simulink model "simulacion2025"  (R2025a)
settings: Solver=VariableStepAuto  StartTime=0.0  StopTime=30  MaxStep=1e-3  RelTol=1e-4
values from neighbouring files (symbols this model uses):
  B = 0.3441    [datos_planta.m]
  Fg = 0.6263    [datos_planta.m]
  J = 0.0112    [datos_planta.m]
  Jb = (305490.04e-12)*0.1    (= 3.0549004e-08)    [datos_planta.m]
  Jv = 13576.379e-12    (= 1.3576379e-08)    [datos_planta.m]
  Ka = 0.2335    [datos_planta.m]
  Km = 0.147    [datos_planta.m]
  L = 0.52    [datos_planta.m]
  m = 0.06385    [datos_planta.m]
  R = 1.6    [datos_planta.m]
  Rr = 21    [datos_planta.m]
  Tm = 0.41    [datos_planta.m]
undefined symbols (not defined in the file or in its folder): x
libraries: slpidlib x31
(part 2 of 2)

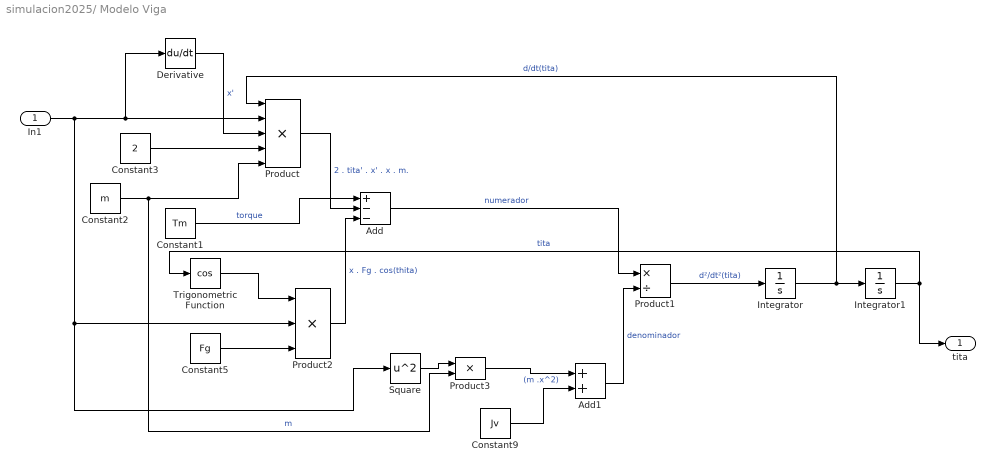
== system simulacion2025/ Modelo Viga ==
  In1 : Inport
  Add : Sum  Inputs=+--
  Add1 : Sum
  Constant1 : Constant  Value=Tm
  Constant2 : Constant  Value=m
  Constant3 : Constant  Value=2
  Constant5 : Constant  Value=Fg
  Constant9 : Constant  Value=Jv
  Derivative : Derivative
  Integrator : Integrator
  Integrator1 : Integrator
  Product : Product  Inputs=5
  Product1 : Product  Inputs=*/
  Product2 : Product  Inputs=3
  Product3 : Product
  Square : Math  Operator=square
  Trigonometric Function : Trigonometry  Operator=cos
  tita : Outport
  wires:
  Product1/1 -> Integrator/1  "d²/dt²(tita)"
  Integrator1/1 -> tita/1, Trigonometric Function/1  "tita"
  Integrator/1 -> Product/1, Integrator1/1  "d/dt(tita)"
  Product/1 -> Add/2  "2 . tita' . x' . x . m."
  Constant2/1 -> Product3/2, Product/5  "m"
  Constant3/1 -> Product/4
  Derivative/1 -> Product/3  "x'"
  Trigonometric Function/1 -> Product2/1
  In1/1 -> Product2/2, Square/1, Derivative/1, Product/2
  Constant5/1 -> Product2/3
  Product2/1 -> Add/3  "x . Fg . cos(thita)"
  Add/1 -> Product1/1  "numerador"
  Constant1/1 -> Add/1  "torque"
  Square/1 -> Product3/1
  Product3/1 -> Add1/1  "(m .x^2)"
  Add1/1 -> Product1/2  "denominador"
  Constant9/1 -> Add1/2

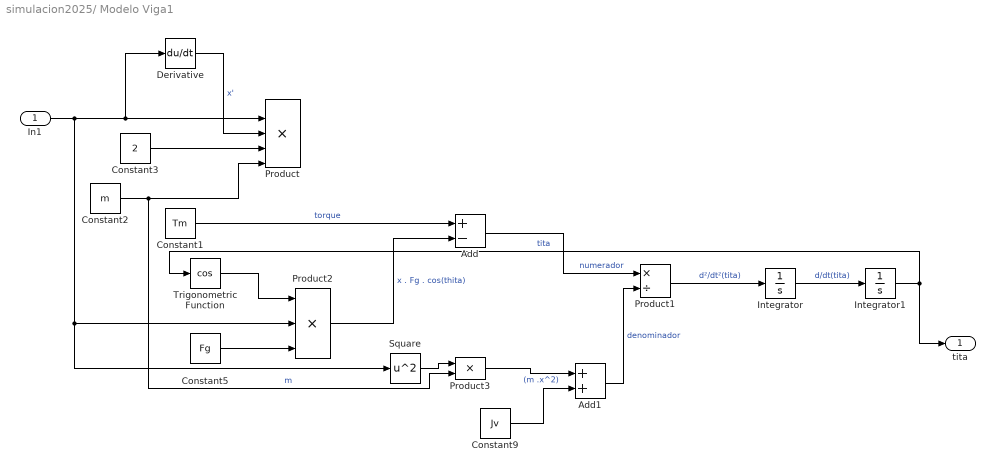
== system simulacion2025/ Modelo Viga1 ==
  In1 : Inport
  Add : Sum  Inputs=+-
  Add1 : Sum
  Constant1 : Constant  Value=Tm
  Constant2 : Constant  Value=m
  Constant3 : Constant  Value=2
  Constant5 : Constant  Value=Fg
  Constant9 : Constant  Value=Jv
  Derivative : Derivative
  Integrator : Integrator
  Integrator1 : Integrator
  Product : Product  Inputs=5
  Product1 : Product  Inputs=*/
  Product2 : Product  Inputs=3
  Product3 : Product
  Square : Math  Operator=square
  Trigonometric Function : Trigonometry  Operator=cos
  tita : Outport
  wires:
  Product1/1 -> Integrator/1  "d²/dt²(tita)"
  Integrator1/1 -> tita/1, Trigonometric Function/1  "tita"
  Integrator/1 -> Integrator1/1  "d/dt(tita)"
  Constant2/1 -> Product3/2, Product/5  "m"
  Constant3/1 -> Product/4
  Derivative/1 -> Product/3  "x'"
  Trigonometric Function/1 -> Product2/1
  In1/1 -> Product2/2, Square/1, Derivative/1, Product/2
  Constant5/1 -> Product2/3
  Constant1/1 -> Add/1  "torque"
  Square/1 -> Product3/1
  Product3/1 -> Add1/1  "(m .x^2)"
  Add1/1 -> Product1/2  "denominador"
  Constant9/1 -> Add1/2
  Product2/1 -> Add/2  "x . Fg . cos(thita)"
  Add/1 -> Product1/1  "numerador"

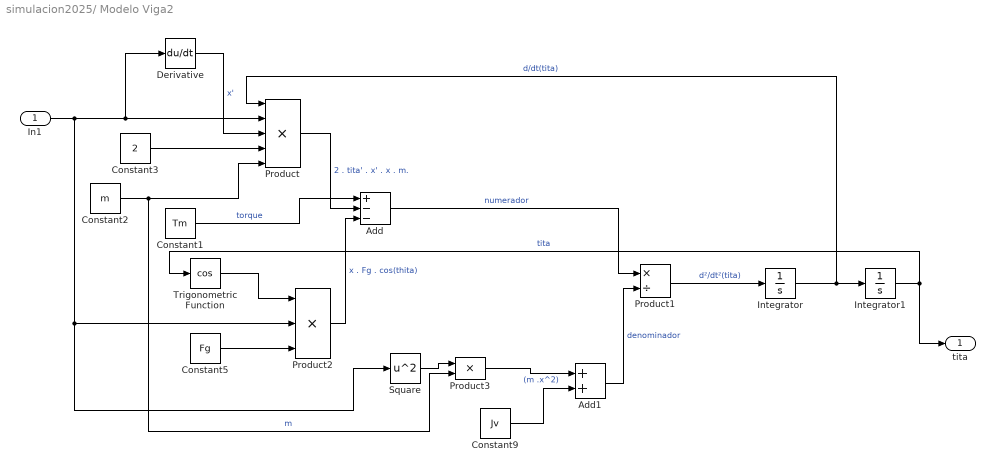
== system simulacion2025/ Modelo Viga2 ==
  In1 : Inport
  Add : Sum  Inputs=+--
  Add1 : Sum
  Constant1 : Constant  Value=Tm
  Constant2 : Constant  Value=m
  Constant3 : Constant  Value=2
  Constant5 : Constant  Value=Fg
  Constant9 : Constant  Value=Jv
  Derivative : Derivative
  Integrator : Integrator
  Integrator1 : Integrator
  Product : Product  Inputs=5
  Product1 : Product  Inputs=*/
  Product2 : Product  Inputs=3
  Product3 : Product
  Square : Math  Operator=square
  Trigonometric Function : Trigonometry  Operator=cos
  tita : Outport
  wires:
  Product1/1 -> Integrator/1  "d²/dt²(tita)"
  Integrator1/1 -> tita/1, Trigonometric Function/1  "tita"
  Integrator/1 -> Product/1, Integrator1/1  "d/dt(tita)"
  Product/1 -> Add/2  "2 . tita' . x' . x . m."
  Constant2/1 -> Product3/2, Product/5  "m"
  Constant3/1 -> Product/4
  Derivative/1 -> Product/3  "x'"
  Trigonometric Function/1 -> Product2/1
  In1/1 -> Product2/2, Square/1, Derivative/1, Product/2
  Constant5/1 -> Product2/3
  Product2/1 -> Add/3  "x . Fg . cos(thita)"
  Add/1 -> Product1/1  "numerador"
  Constant1/1 -> Add/1  "torque"
  Square/1 -> Product3/1
  Product3/1 -> Add1/1  "(m .x^2)"
  Add1/1 -> Product1/2  "denominador"
  Constant9/1 -> Add1/2

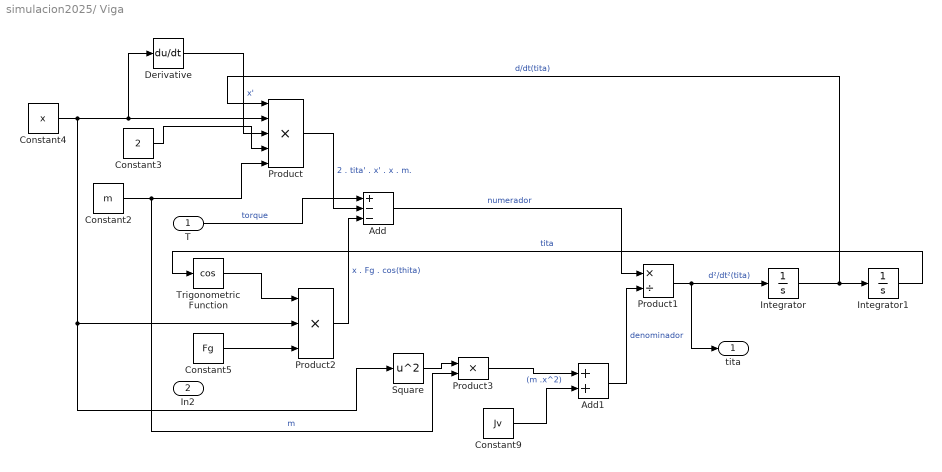
== system simulacion2025/ Viga ==
  T : Inport
  In2 : Inport  Port=2
  Add : Sum  Inputs=+--
  Add1 : Sum
  Constant2 : Constant  Value=m
  Constant3 : Constant  Value=2
  Constant4 : Constant  Value=x
  Constant5 : Constant  Value=Fg
  Constant9 : Constant  Value=Jv
  Derivative : Derivative
  Integrator : Integrator
  Integrator1 : Integrator
  Product : Product  Inputs=5
  Product1 : Product  Inputs=*/
  Product2 : Product  Inputs=3
  Product3 : Product
  Square : Math  Operator=square
  Trigonometric Function : Trigonometry  Operator=cos
  tita : Outport
  wires:
  Product1/1 -> tita/1, Integrator/1  "d²/dt²(tita)"
  Integrator1/1 -> Trigonometric Function/1  "tita"
  Integrator/1 -> Product/1, Integrator1/1  "d/dt(tita)"
  Product/1 -> Add/2  "2 . tita' . x' . x . m."
  Constant2/1 -> Product3/2, Product/5  "m"
  Constant3/1 -> Product/4
  Derivative/1 -> Product/3  "x'"
  Trigonometric Function/1 -> Product2/1
  Constant4/1 -> Product2/2, Square/1, Derivative/1, Product/2
  Constant5/1 -> Product2/3
  Product2/1 -> Add/3  "x . Fg . cos(thita)"
  Add/1 -> Product1/1  "numerador"
  T/1 -> Add/1  "torque"
  Square/1 -> Product3/1
  Product3/1 -> Add1/1  "(m .x^2)"
  Add1/1 -> Product1/2  "denominador"
  Constant9/1 -> Add1/2

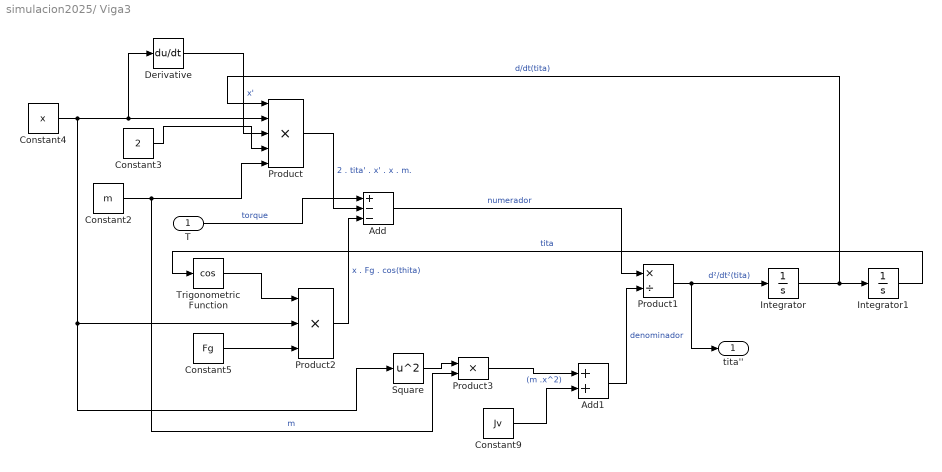
== system simulacion2025/ Viga3 ==
  T : Inport
  Add : Sum  Inputs=+--
  Add1 : Sum
  Constant2 : Constant  Value=m
  Constant3 : Constant  Value=2
  Constant4 : Constant  Value=x
  Constant5 : Constant  Value=Fg
  Constant9 : Constant  Value=Jv
  Derivative : Derivative
  Integrator : Integrator
  Integrator1 : Integrator
  Product : Product  Inputs=5
  Product1 : Product  Inputs=*/
  Product2 : Product  Inputs=3
  Product3 : Product
  Square : Math  Operator=square
  Trigonometric Function : Trigonometry  Operator=cos
  tita'' : Outport
  wires:
  Product1/1 -> tita''/1, Integrator/1  "d²/dt²(tita)"
  Integrator1/1 -> Trigonometric Function/1  "tita"
  Integrator/1 -> Product/1, Integrator1/1  "d/dt(tita)"
  Product/1 -> Add/2  "2 . tita' . x' . x . m."
  Constant2/1 -> Product3/2, Product/5  "m"
  Constant3/1 -> Product/4
  Derivative/1 -> Product/3  "x'"
  Trigonometric Function/1 -> Product2/1
  Constant4/1 -> Product2/2, Square/1, Derivative/1, Product/2
  Constant5/1 -> Product2/3
  Product2/1 -> Add/3  "x . Fg . cos(thita)"
  Add/1 -> Product1/1  "numerador"
  T/1 -> Add/1  "torque"
  Square/1 -> Product3/1
  Product3/1 -> Add1/1  "(m .x^2)"
  Add1/1 -> Product1/2  "denominador"
  Constant9/1 -> Add1/2

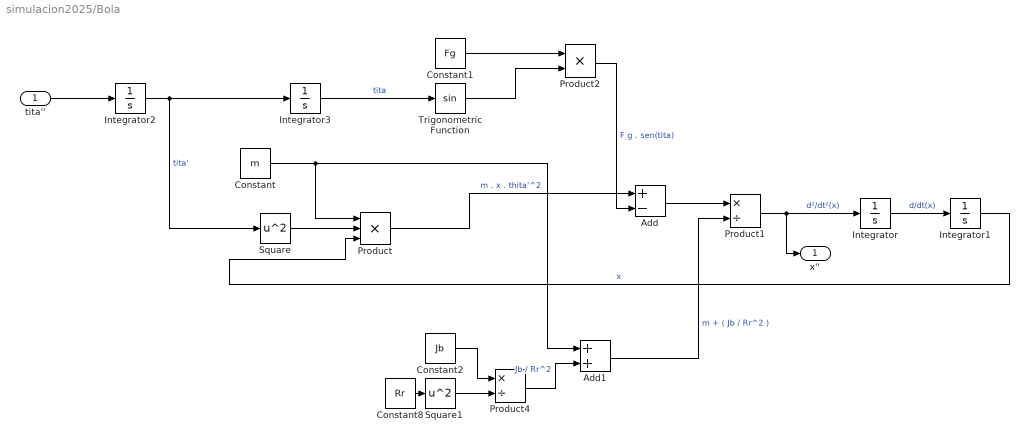
== system simulacion2025/Bola ==
  tita'' : Inport
  Add : Sum  Inputs=+-
  Add1 : Sum
  Constant : Constant  Value=m
  Constant1 : Constant  Value=Fg
  Constant2 : Constant  Value=Jb
  Constant8 : Constant  Value=Rr
  Integrator{,1..3} (4 alike) : Integrator
  Product : Product  Inputs=3
  Product1 : Product  Inputs=*/
  Product2 : Product
  Product4 : Product  Inputs=*/
  Square : Math  Operator=square
  Square1 : Math  Operator=square
  Trigonometric Function : Trigonometry
  x'' : Outport
  wires:
  Add/1 -> Product1/1
  Square/1 -> Product/2
  Integrator/1 -> Integrator1/1  "d/dt(x)"
  Integrator1/1 -> Product/3  "x"
  Integrator2/1 -> Square/1, Integrator3/1  "tita'"
  Product/1 -> Add/1  "m . x . thita'^2"
  Constant1/1 -> Product2/1
  Product2/1 -> Add/2  "F g . sen(tita)"
  tita''/1 -> Integrator2/1
  Product1/1 -> x''/1, Integrator/1  "d²/dt²(x)"
  Product4/1 -> Add1/2  "Jb / Rr^2"
  Constant2/1 -> Product4/1
  Constant/1 -> Add1/1, Product/1
  Square1/1 -> Product4/2
  Constant8/1 -> Square1/1
  Add1/1 -> Product1/2  "m + ( Jb / Rr^2 )"
  Integrator3/1 -> Trigonometric Function/1  "tita"
  Trigonometric Function/1 -> Product2/2

== system simulacion2025/Bola PosTaylor1 ==
  Constant2 : Constant  Value=Jb
  Constant6 : Constant  Value=-Fg
  Constant7 : Constant  Value=m
  Constant8 : Constant  Value=Rr
  Integrator1 : Integrator
  Integrator5 : Integrator
  Minus1 : Sum
  Product4 : Product  Inputs=*/
  Product7 : Product  Inputs=*/
  Square1 : Math  Operator=square
  Out1 : Outport
  wires:
  Constant6/1 -> Product7/1  "-Fg"
  Product7/1 -> Integrator5/1  "d²/dt²(x)"
  Integrator5/1 -> Integrator1/1  "delta.d(x)/dt"
  Integrator1/1 -> Out1/1  "d/dt(x)"
  Constant2/1 -> Product4/1
  Square1/1 -> Product4/2
  Constant8/1 -> Square1/1
  Product4/1 -> Minus1/2
  Constant7/1 -> Minus1/1
  Minus1/1 -> Product7/2

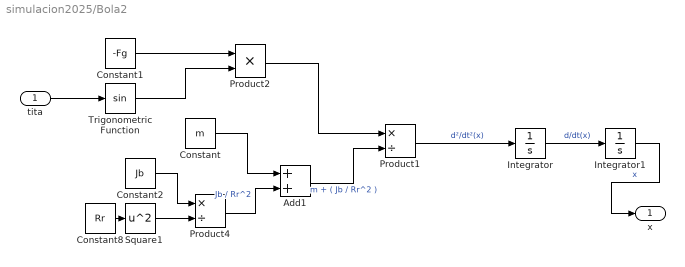
== system simulacion2025/Bola2 ==
  tita : Inport
  Add1 : Sum
  Constant : Constant  Value=m
  Constant1 : Constant  Value=-Fg
  Constant2 : Constant  Value=Jb
  Constant8 : Constant  Value=Rr
  Integrator : Integrator
  Integrator1 : Integrator
  Product1 : Product  Inputs=*/
  Product2 : Product
  Product4 : Product  Inputs=*/
  Square1 : Math  Operator=square
  Trigonometric Function : Trigonometry
  x : Outport
  wires:
  Product2/1 -> Product1/1
  Integrator/1 -> Integrator1/1  "d/dt(x)"
  Constant1/1 -> Product2/1
  Product1/1 -> Integrator/1  "d²/dt²(x)"
  Product4/1 -> Add1/2  "Jb / Rr^2"
  Constant2/1 -> Product4/1
  Constant/1 -> Add1/1
  Square1/1 -> Product4/2
  Constant8/1 -> Square1/1
  Add1/1 -> Product1/2  "m + ( Jb / Rr^2 )"
  tita/1 -> Trigonometric Function/1
  Trigonometric Function/1 -> Product2/2
  Integrator1/1 -> x/1  "x"

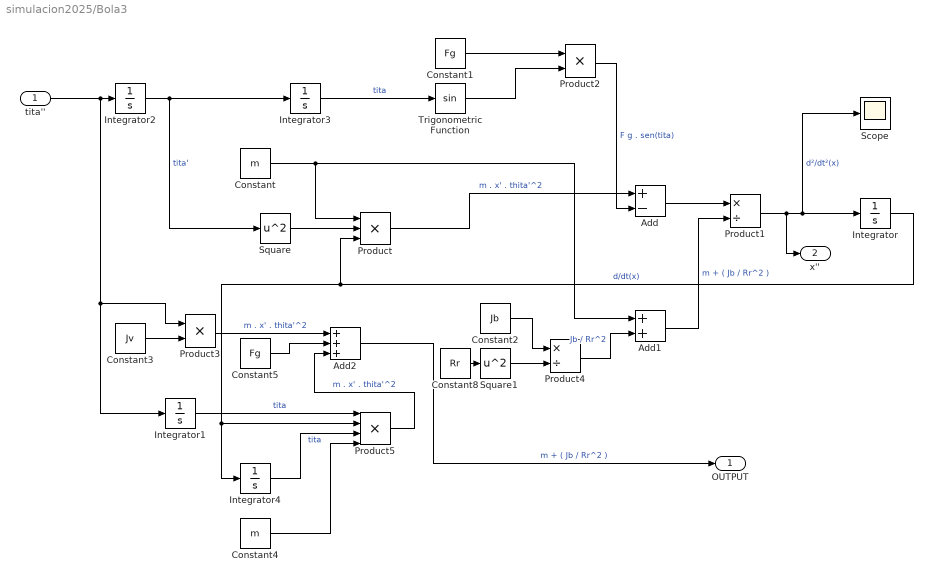
== system simulacion2025/Bola3 ==
  tita'' : Inport
  Add : Sum  Inputs=+-
  Add1 : Sum
  Add2 : Sum  Inputs=+++
  Constant : Constant  Value=m
  Constant1 : Constant  Value=Fg
  Constant2 : Constant  Value=Jb
  Constant3 : Constant  Value=Jv
  Constant4 : Constant  Value=m
  Constant5 : Constant  Value=Fg
  Constant8 : Constant  Value=Rr
  Integrator{,1..4} (5 alike) : Integrator
  Product : Product  Inputs=3
  Product1 : Product  Inputs=*/
  Product2 : Product
  Product3 : Product
  Product4 : Product  Inputs=*/
  Product5 : Product  Inputs=4
  Scope : Scope
      settings: ActiveDisplayYMinimum=-1.4787523574592083E+300  ActiveDisplayYMaximum=1.3308771217132878E+301  DataLoggingVariableName=ScopeData2
  Square : Math  Operator=square
  Square1 : Math  Operator=square
  Trigonometric Function : Trigonometry
  OUTPUT : Outport
  x'' : Outport  Port=2
  wires:
  Add/1 -> Product1/1
  Square/1 -> Product/2
  Integrator/1 -> Integrator4/1, Product5/2, Product/3  "d/dt(x)"
  Integrator2/1 -> Square/1, Integrator3/1  "tita'"
  Product/1 -> Add/1  "m . x' . thita'^2"
  Constant1/1 -> Product2/1
  Product2/1 -> Add/2  "F g . sen(tita)"
  Product1/1 -> x''/1, Scope/1, Integrator/1  "d²/dt²(x)"
  Product4/1 -> Add1/2  "Jb / Rr^2"
  Constant2/1 -> Product4/1
  Constant/1 -> Add1/1, Product/1
  Square1/1 -> Product4/2
  Constant8/1 -> Square1/1
  Add1/1 -> Product1/2  "m + ( Jb / Rr^2 )"
  Integrator3/1 -> Trigonometric Function/1  "tita"
  Trigonometric Function/1 -> Product2/2
  tita''/1 -> Integrator1/1, Product3/1, Integrator2/1
  Constant3/1 -> Product3/2
  Product3/1 -> Add2/1  "m . x' . thita'^2"
  Integrator1/1 -> Product5/1  "tita"
  Integrator4/1 -> Product5/3  "tita"
  Constant4/1 -> Product5/4
  Add2/1 -> OUTPUT/1  "m + ( Jb / Rr^2 )"
  Product5/1 -> Add2/3  "m . x' . thita'^2"
  Constant5/1 -> Add2/2

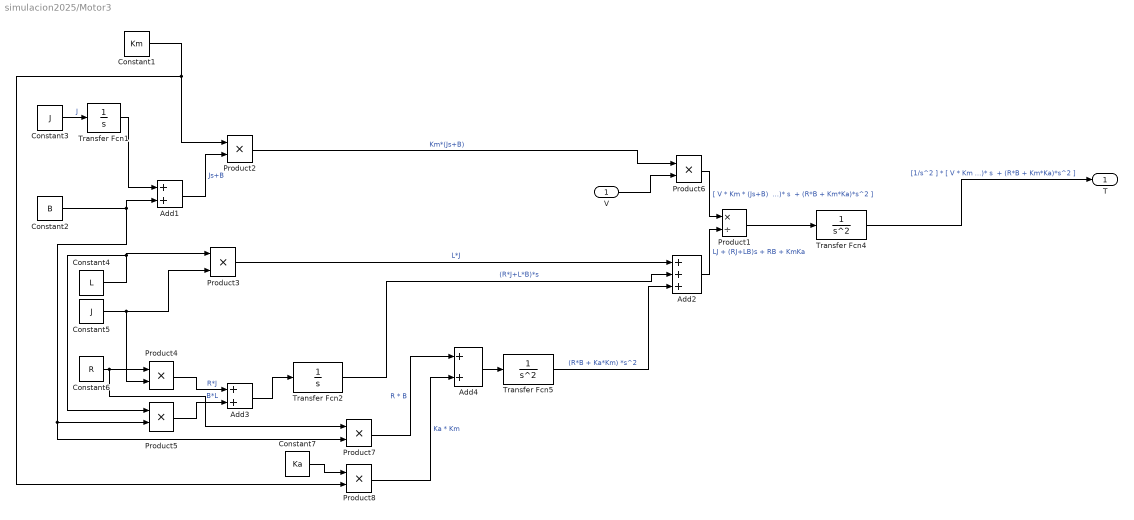
== system simulacion2025/Motor3 ==
  V : Inport
  Add1 : Sum
  Add2 : Sum  Inputs=+++
  Add3 : Sum
  Add4 : Sum
  Constant1 : Constant  Value=Km
  Constant2 : Constant  Value=B
  Constant3 : Constant  Value=J
  Constant4 : Constant  Value=L
  Constant5 : Constant  Value=J
  Constant6 : Constant  Value=R
  Constant7 : Constant  Value=Ka
  Product1 : Product  Inputs=*/
  Product{2..8} (7 alike) : Product
  Transfer Fcn1 : TransferFcn  Denominator=[0 1 0]
  Transfer Fcn2 : TransferFcn  Denominator=[0 1 0]
  Transfer Fcn4 : TransferFcn  Denominator=[1 0 0]
  Transfer Fcn5 : TransferFcn  Denominator=[1 0 0]
  T : Outport
  wires:
  Add1/1 -> Product2/2  "Js+B"
  Product2/1 -> Product6/1  "Km*(Js+B)"
  Constant5/1 -> Product3/2, Product4/2
  Constant4/1 -> Product5/1, Product3/1
  Product4/1 -> Add3/1  "R*J"
  Product5/1 -> Add3/2  "B*L"
  Add2/1 -> Product1/2  "LJ + (RJ+LB)s + RB + KmKa"
  Add3/1 -> Transfer Fcn2/1
  Transfer Fcn2/1 -> Add2/2  "(R*J+L*B)*s"
  Constant6/1 -> Product7/1, Product4/1
  Constant2/1 -> Add1/2, Product7/2, Product5/2
  Product7/1 -> Add4/1  "R * B"
  Constant7/1 -> Product8/1
  Constant1/1 -> Product2/1, Product8/2
  Product8/1 -> Add4/2  "Ka * Km"
  Constant3/1 -> Transfer Fcn1/1  "J"
  Product3/1 -> Add2/1  "L*J"
  Transfer Fcn4/1 -> T/1  "[1/s^2 ] * [ V * Km * (Js+B)  /  L*J + (RJ+LB)* s  + (R*B + Km*Ka)*s^2 ]"
  V/1 -> Product6/2
  Product6/1 -> Product1/1  "[ V * Km * (Js+B)  /  L*J + (RJ+LB)* s  + (R*B + Km*Ka)*s^2 ]"
  Product1/1 -> Transfer Fcn4/1
  Add4/1 -> Transfer Fcn5/1
  Transfer Fcn5/1 -> Add2/3  "(R*B + Ka*Km) *s^2"
  Transfer Fcn1/1 -> Add1/1

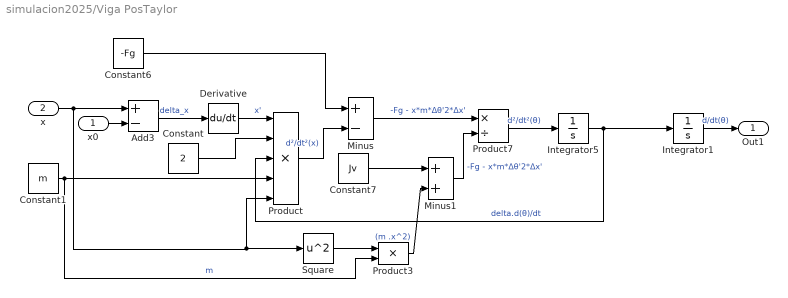
== system simulacion2025/Viga PosTaylor ==
  x0 : Inport
  x : Inport  Port=2
  Add3 : Sum  Inputs=+-
  Constant : Constant  Value=2
  Constant1 : Constant  Value=m
  Constant6 : Constant  Value=-Fg
  Constant7 : Constant  Value=Jv
  Derivative : Derivative
  Integrator1 : Integrator
  Integrator5 : Integrator
  Minus : Sum  Inputs=+-
  Minus1 : Sum
  Product : Product  Inputs=5
  Product3 : Product
  Product7 : Product  Inputs=*/
  Square : Math  Operator=square
  Out1 : Outport
  wires:
  x0/1 -> Add3/2
  Minus/1 -> Product7/1  "-Fg - x*m*Δθ'2*Δx'"
  Product7/1 -> Integrator5/1  "d²/dt²(θ)"
  Integrator5/1 -> Product/3, Integrator1/1  "delta.d(θ)/dt"
  Constant6/1 -> Minus/1
  Add3/1 -> Derivative/1  "delta_x"
  Product/1 -> Minus/2  "d²/dt²(x)"
  Derivative/1 -> Product/1  "x'"
  Constant/1 -> Product/2
  Integrator1/1 -> Out1/1  "d/dt(θ)"
  Constant1/1 -> Product/4, Product3/2  "m"
  Square/1 -> Product3/1
  x/1 -> Add3/1, Square/1, Product/5
  Constant7/1 -> Minus1/1
  Product3/1 -> Minus1/2  "(m .x^2)"
  Minus1/1 -> Product7/2  "-Fg - x*m*Δθ'2*Δx'"

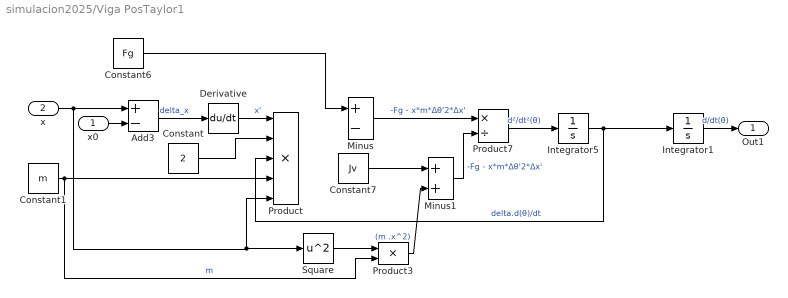
== system simulacion2025/Viga PosTaylor1 ==
  x0 : Inport
  x : Inport  Port=2
  Add3 : Sum  Inputs=+-
  Constant : Constant  Value=2
  Constant1 : Constant  Value=m
  Constant6 : Constant  Value=Fg
  Constant7 : Constant  Value=Jv
  Derivative : Derivative
  Integrator1 : Integrator
  Integrator5 : Integrator
  Minus : Sum  Inputs=+-
  Minus1 : Sum
  Product : Product  Inputs=5
  Product3 : Product
  Product7 : Product  Inputs=*/
  Square : Math  Operator=square
  Out1 : Outport
  wires:
  x0/1 -> Add3/2
  Minus/1 -> Product7/1  "-Fg - x*m*Δθ'2*Δx'"
  Product7/1 -> Integrator5/1  "d²/dt²(θ)"
  Integrator5/1 -> Product/3, Integrator1/1  "delta.d(θ)/dt"
  Constant6/1 -> Minus/1
  Add3/1 -> Derivative/1  "delta_x"
  Derivative/1 -> Product/1  "x'"
  Constant/1 -> Product/2
  Integrator1/1 -> Out1/1  "d/dt(θ)"
  Constant1/1 -> Product/4, Product3/2  "m"
  Square/1 -> Product3/1
  x/1 -> Add3/1, Square/1, Product/5
  Product3/1 -> Minus1/2  "(m .x^2)"
  Constant7/1 -> Minus1/1
  Minus1/1 -> Product7/2  "-Fg - x*m*Δθ'2*Δx'"
